simulink model "mpc_active_suspension_2020b"  (R2020b)
settings: Solver=FixedStepAuto  StartTime=0.0  StopTime=10  FixedStep=0.001  MaxStep=0.001  RelTol=1e-3
undefined symbols (not defined in the file): A, B, C, D, kw, Q, R, sigbuilder_block, T
libraries: simulink x1, dsparch4 x1
settings Model: Creator=ku53058  LastModifiedBy=11508
settings DataIOCC: ReturnWorkspaceOutputs=off
settings OptimizationCC: LifeSpan=inf
settings DebuggingCC: ArithmeticOperatorsInVariantConditions=warning
settings SFSimCC: SimUseLocalCustomCode=off  CustomCodeUndefinedFunction=UseInterfaceOnly
settings RTWCC: RTWUseLocalCustomCode=off
settings CodeAppCC: StateflowObjectComments=on

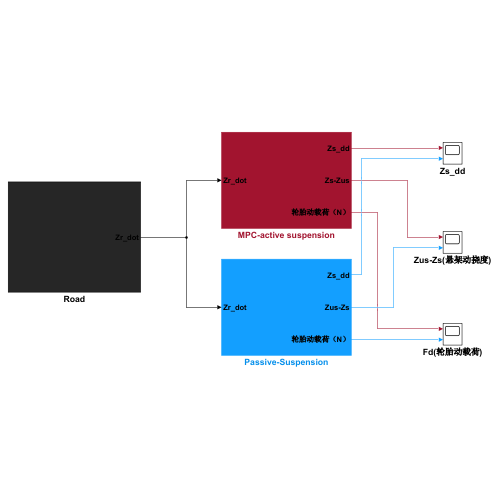
[thumbnail: Simulink's stored preview of the top-level diagram]
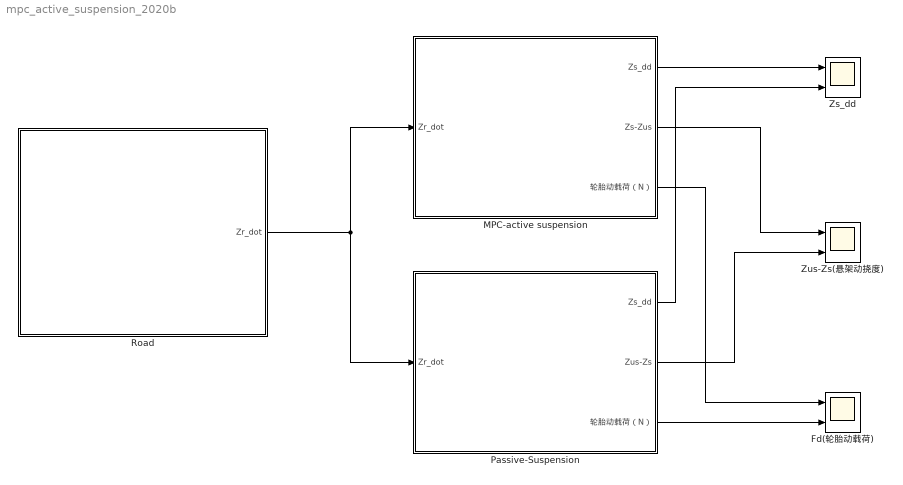
== system mpc_active_suspension_2020b ==
  Fd(轮胎动载荷) : Scope  NumInputPorts=2
  MPC-active suspension : Subsystem
  Passive-Suspension : Subsystem
  Road : Subsystem
  Zs_dd : Scope  NumInputPorts=2
  Zus-Zs(悬架动挠度) : Scope  NumInputPorts=2
  wires:
  MPC-active suspension/3(轮胎动载荷（N）) -> Fd(轮胎动载荷)/1
  MPC-active suspension/2(Zs-Zus) -> Zus-Zs(悬架动挠度)/1
  Road/1(Zr_dot) -> MPC-active suspension/1(Zr_dot), Passive-Suspension/1(Zr_dot)
  MPC-active suspension/1(Zs_dd) -> Zs_dd/1
  Passive-Suspension/3(轮胎动载荷（N）) -> Fd(轮胎动载荷)/2
  Passive-Suspension/2(Zus-Zs) -> Zus-Zs(悬架动挠度)/2
  Passive-Suspension/1(Zs_dd) -> Zs_dd/2

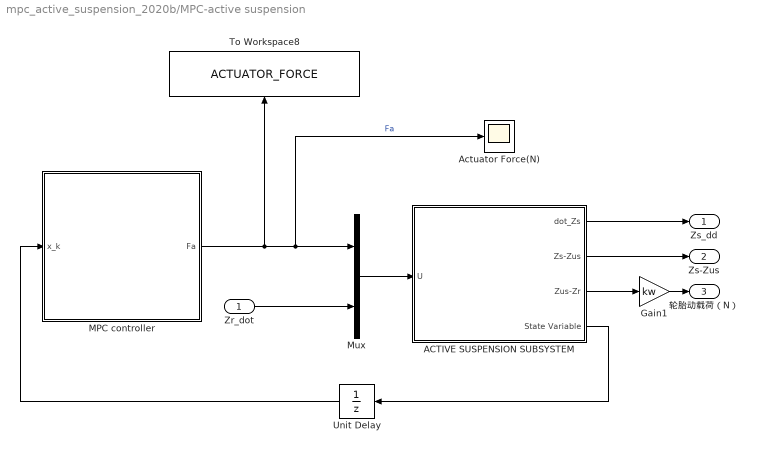
== system mpc_active_suspension_2020b/MPC-active suspension ==
  Zr_dot : Inport
  ACTIVE SUSPENSION SUBSYSTEM : Subsystem
  Actuator Force(N) : Scope
  Gain1 : Gain  Gain=kw
  MPC controller : Subsystem
  Mux : Mux  Inputs=2
  To Workspace8 : ToWorkspace  VariableName=ACTUATOR_FORCE  SampleTime=-1
  Unit Delay : UnitDelay  SampleTime=-1  HasFrameUpgradeWarning=on
  Zs_dd : Outport
  Zs-Zus : Outport  Port=2
  轮胎动载荷（N） : Outport  Port=3
  wires:
  Mux/1 -> ACTIVE SUSPENSION SUBSYSTEM/1(U)
  MPC controller/1(Fa) -> Mux/1, Actuator Force(N)/1, To Workspace8/1  "Fa"
  ACTIVE SUSPENSION SUBSYSTEM/2(Zs-Zus) -> Zs-Zus/1
  ACTIVE SUSPENSION SUBSYSTEM/3(Zus-Zr) -> Gain1/1
  Gain1/1 -> 轮胎动载荷（N）/1
  ACTIVE SUSPENSION SUBSYSTEM/1(dot_Zs) -> Zs_dd/1
  Zr_dot/1 -> Mux/2
  ACTIVE SUSPENSION SUBSYSTEM/4(State Variable) -> Unit Delay/1
  Unit Delay/1 -> MPC controller/1(x_k)

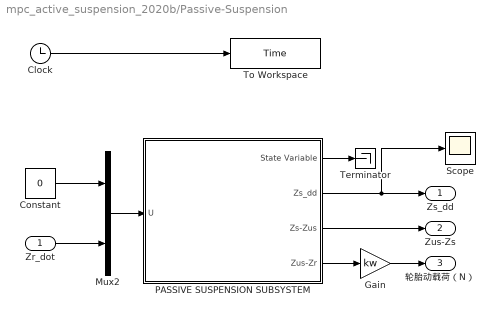
== system mpc_active_suspension_2020b/Passive-Suspension ==
  Zr_dot : Inport
  Clock : Clock
  Constant : Constant  Value=0
  Gain : Gain  Gain=kw
  Mux2 : Mux  Inputs=2
  PASSIVE SUSPENSION SUBSYSTEM : Subsystem
  Scope : Scope
  Terminator : Terminator
  To Workspace : ToWorkspace  VariableName=Time  SampleTime=-1
  Zs_dd : Outport
  Zus-Zs : Outport  Port=2
  轮胎动载荷（N） : Outport  Port=3
  wires:
  Mux2/1 -> PASSIVE SUSPENSION SUBSYSTEM/1(U)
  PASSIVE SUSPENSION SUBSYSTEM/3(Zs-Zus) -> Zus-Zs/1
  PASSIVE SUSPENSION SUBSYSTEM/2(Zs_dd) -> Scope/1, Zs_dd/1
  Gain/1 -> 轮胎动载荷（N）/1
  PASSIVE SUSPENSION SUBSYSTEM/4(Zus-Zr) -> Gain/1
  Zr_dot/1 -> Mux2/2
  Constant/1 -> Mux2/1
  Clock/1 -> To Workspace/1
  PASSIVE SUSPENSION SUBSYSTEM/1(State Variable) -> Terminator/1

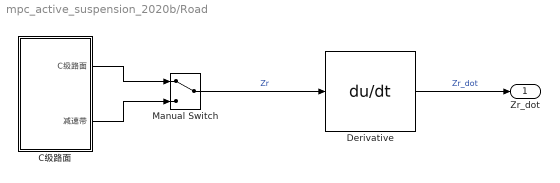
== system mpc_active_suspension_2020b/Road ==
  C级路面 : Subsystem
  Derivative : Derivative
  Manual Switch : ManualSwitch
  Zr_dot : Outport
  wires:
  Manual Switch/1 -> Derivative/1  "Zr"
  Derivative/1 -> Zr_dot/1  "Zr_dot"
  C级路面/2(减速带) -> Manual Switch/2
  C级路面/1(C级路面) -> Manual Switch/1

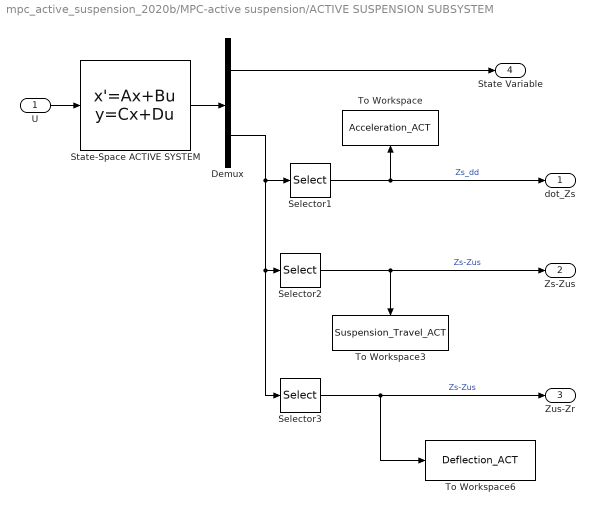
== system mpc_active_suspension_2020b/MPC-active suspension/ACTIVE SUSPENSION SUBSYSTEM ==
  U : Inport
  Demux : Demux  Outputs=[4 3]
  Selector1 : Selector  InputPortWidth=3  IndexOptions=Index vector (dialog)  Indices=[1]  OutputSizes=1
  Selector2 : Selector  InputPortWidth=3  IndexOptions=Index vector (dialog)  Indices=2  OutputSizes=1
  Selector3 : Selector  InputPortWidth=3  IndexOptions=Index vector (dialog)  Indices=3  OutputSizes=1
  State-Space ACTIVE SYSTEM : StateSpace  A=A  B=cat(2,B,E)  C=cat(1,eye(4), C)  D=cat(1,zeros(4,2),cat(2,D,T))  InitialCondition=0
  To Workspace : ToWorkspace  VariableName=Acceleration_ACT  SampleTime=-1
  To Workspace3 : ToWorkspace  VariableName=Suspension_Travel_ACT  SampleTime=-1
  To Workspace6 : ToWorkspace  VariableName=Deflection_ACT  SampleTime=-1
  dot_Zs : Outport
  Zs-Zus : Outport  Port=2
  Zus-Zr : Outport  Port=3
  State Variable : Outport  Port=4
  wires:
  Demux/1 -> State Variable/1
  State-Space ACTIVE SYSTEM/1 -> Demux/1
  Demux/2 -> Selector1/1, Selector3/1, Selector2/1
  Selector1/1 -> dot_Zs/1, To Workspace/1  "Zs_dd"
  Selector2/1 -> Zs-Zus/1, To Workspace3/1  "Zs-Zus"
  U/1 -> State-Space ACTIVE SYSTEM/1
  Selector3/1 -> To Workspace6/1, Zus-Zr/1  "Zs-Zus"

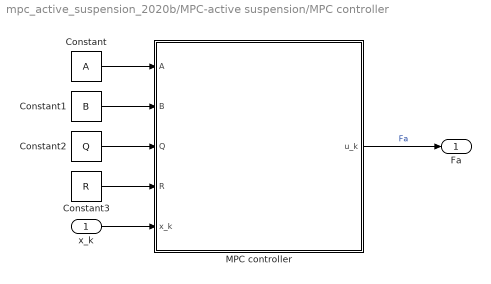
== system mpc_active_suspension_2020b/MPC-active suspension/MPC controller ==
  x_k : Inport
  Constant : Constant  Value=A  VectorParams1D=off
  Constant1 : Constant  Value=B  VectorParams1D=off
  Constant2 : Constant  Value=Q  VectorParams1D=off
  Constant3 : Constant  Value=R  VectorParams1D=off
  MPC controller : MATLAB Function  TreatAsAtomicUnit=on
  Fa : Outport
  wires:
  Constant/1 -> MPC controller/1(A)
  Constant2/1 -> MPC controller/3(Q)
  Constant3/1 -> MPC controller/4(R)
  x_k/1 -> MPC controller/5(x_k)
  Constant1/1 -> MPC controller/2(B)
  MPC controller/1(u_k) -> Fa/1  "Fa"

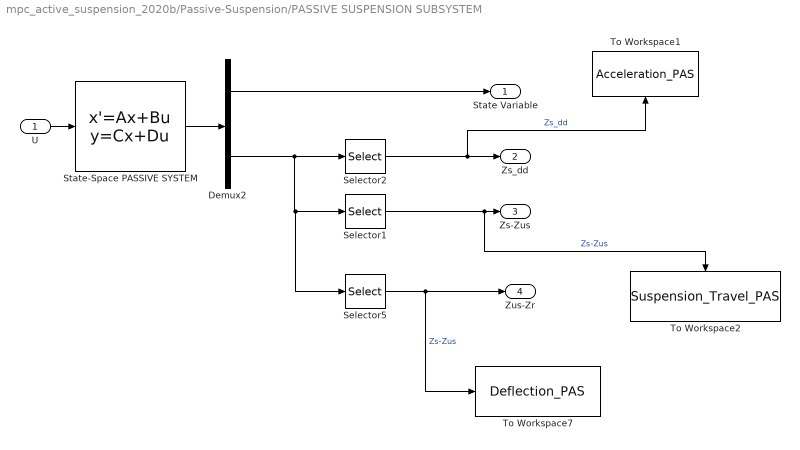
== system mpc_active_suspension_2020b/Passive-Suspension/PASSIVE SUSPENSION SUBSYSTEM ==
  U : Inport
  Demux2 : Demux  Outputs=[4 3]
  Selector1 : Selector  InputPortWidth=3  IndexOptions=Index vector (dialog)  Indices=2  OutputSizes=1
  Selector2 : Selector  InputPortWidth=3  IndexOptions=Index vector (dialog)  Indices=[1]  OutputSizes=1
  Selector5 : Selector  InputPortWidth=3  IndexOptions=Index vector (dialog)  Indices=3  OutputSizes=1
  State-Space PASSIVE SYSTEM : StateSpace  A=A  B=cat(2,B,E)  C=cat(1,eye(4), C)  D=cat(1,zeros(4,2),cat(2,D,T))  InitialCondition=0
  To Workspace1 : ToWorkspace  VariableName=Acceleration_PAS  SampleTime=-1
  To Workspace2 : ToWorkspace  VariableName=Suspension_Travel_PAS  SampleTime=-1
  To Workspace7 : ToWorkspace  VariableName=Deflection_PAS  SampleTime=-1
  State Variable : Outport
  Zs_dd : Outport  Port=2
  Zs-Zus : Outport  Port=3
  Zus-Zr : Outport  Port=4
  wires:
  State-Space PASSIVE SYSTEM/1 -> Demux2/1
  U/1 -> State-Space PASSIVE SYSTEM/1
  Demux2/1 -> State Variable/1
  Demux2/2 -> Selector5/1, Selector1/1, Selector2/1
  Selector2/1 -> To Workspace1/1, Zs_dd/1  "Zs_dd"
  Selector1/1 -> Zs-Zus/1, To Workspace2/1  "Zs-Zus"
  Selector5/1 -> To Workspace7/1, Zus-Zr/1  "Zs-Zus"

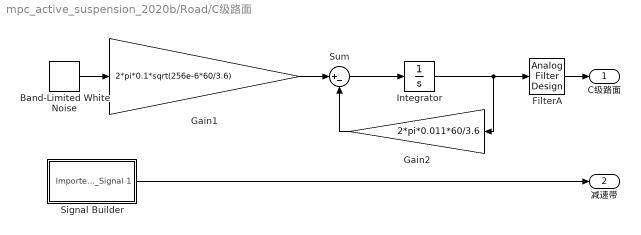
== system mpc_active_suspension_2020b/Road/C级路面 ==
  Band-Limited White Noise : simulink/Sources/Band-Limited White Noise  Cov=0.5  Ts=0.01  seed=[23341]
  FilterA : dsparch4/Analog Filter Design  method=Butterworth  filttype=Bandpass  N=4  Wlo=0.01*2*pi  Whi=20*2*pi  Rp=2  Rs=40
  Gain1 : Gain  Gain=2*pi*0.1*sqrt(256e-6*60/3.6)
  Gain2 : Gain  Gain=2*pi*0.011*60/3.6
  Integrator : Integrator
  Signal Builder : Subsystem  Tag=STV Subsys  LoadFcn=sigbuilder_block('load');  StartFcn=sigbuilder_block('start');  StopFcn=sigbuilder_block('stop');  ClipboardFcn=sigbuilder_block('clipboard');  mask(Sigbuilder block){tuvar=[0:10]}
      mask help: Simulink:masks:SigbuilderBlock_MD
      mask init:
      | if ~strcmp(get_param(bdroot(gcbh),'SimulationStatus'),'stopped') tuvar = sigbuilder_block('maskInit'); end
      settings: CopyFcn=sigbuilder_block('copy');  DeleteFcn=sigbuilder_block('delete');  ModelCloseFcn=sigbuilder_block('modelClose');  PreSaveFcn=sigbuilder_block('preSave');  PauseFcn=sigbuilder_block('pause');  ContinueFcn=sigbuilder_block('continue');  NameChangeFcn=sigbuilder_block('namechange');  OpenFcn=sigbuilder_block('open',[476.5 112.5 550.5 400 ]);  CloseFcn=sigbuilder_block('close');
      mask Display: plot(0, 0, 100, 100,[2, 2, 32, 32, 2], [68, 8, 8, 68, 68],[32, 2], [38, 38], [32, 19, 2],[53, 60, 44], [32, 17, 17, 2],[16, 16, 31, 31]);txt = getActiveGroup(gcbh);text(2, 100, txt,'verticalAlignment', 'top');
  Sum : Sum  Inputs=|+-
  C级路面 : Outport  VectorParamsAs1DForOutWhenUnconnected=off
  减速带 : Outport  Port=2  VectorParamsAs1DForOutWhenUnconnected=off
  wires:
  Signal Builder/1(Imported_Signal 1) -> 减速带/1
  Gain1/1 -> Sum/1
  Sum/1 -> Integrator/1
  Band-Limited White Noise/1 -> Gain1/1
  Integrator/1 -> Gain2/1, FilterA/1
  Gain2/1 -> Sum/2
  FilterA/1 -> C级路面/1

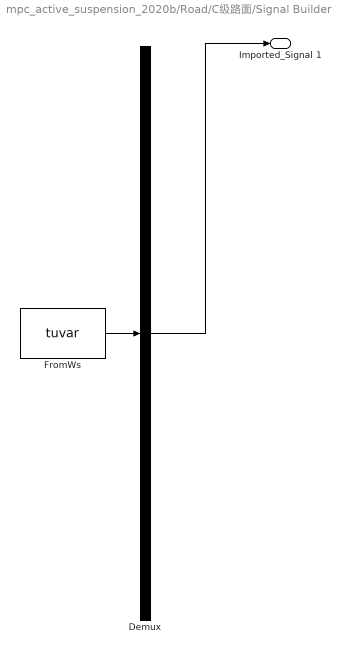
== system mpc_active_suspension_2020b/Road/C级路面/Signal Builder ==
  Demux : Demux  Tag=STV Demux  Outputs=1
      settings: DisplayOption=none
  FromWs : FromWorkspace  Tag=STV FromWs  VariableName=tuvar
      SigBuilderData=|
      | common.afterFinalStr = 'Extrapolate'
      | common.sampleTime = 0
      | dataSet.timeRange = [0 4]
      | dataSet.name = 'Sheet1'
      | sbobj.Groups.Name = 'Sheet1'
      | sbobj.Groups.Signals.Name = 'Imported_Signal 1'
      | sbobj.Groups.Signals.XData = [0 0.001 0.002 0.003 0.004 0.005 0.006 0.007 0.008 0.009 0.01 0.011 ... (4001 elements, 1x4001)]
      | sbobj.Groups.Signals.YData = [0 0 0 0 0 0 0 0 0 0 0 0 ... (4001 elements, 1x4001)]
      | sbobj.Groups.TimeRange = [0 4]
  Imported_Signal 1 : Outport  Tag=STV Outport  VectorParamsAs1DForOutWhenUnconnected=off
  wires:
  Demux/1 -> Imported_Signal 1/1
  FromWs/1 -> Demux/1

== matlab function mpc_active_suspension_2020b/MPC-active suspension/MPC controller/MPC controller ==
  data: A input; B input; Q input; R input; x_k input; u_k output
function u_k= fcn(A,B,Q,R,x_k)
n=size(A,1);   % A 是 n x n 矩阵, 得到 n
dt = 0.001;
I=eye(n);
A1 = I+A*dt;%离散化
B1 = dt*B;
p=size(B1,2);   % B 是 n x p 矩阵, 得到 p
Np = 10; %预测区间
[E,H]=MPC_Matrices(A1,B1,Q,R,Np,n,p); %求得E H矩阵
% 计算
u_k = Prediction(x_k,E,H,Np,p); %求得此步得uk


function  [E,H]=MPC_Matrices(A,B,Q,R,Np,n,p)  %算出E和H矩阵
B_hat=zeros(Np*n,Np*p); % 初始化 B_hat 矩阵, 这一步令它有 Np*n x Np*p 个 0
B_hat(1:n,1:p)=B; %
A_hat = A;
temp = A;
for i =1:(Np-1)  
rows = i*n+(1:n);  % 表示行 i = 1 -> row = n+1 : 2n  那 i = 1 : (Np-1) 行则 n+1 :  (Np-1)n + 1 : Np*n 
B_hat(rows,:)=[temp*B,B_hat(rows-n,1:end-p)]; %temp=A^i,  tempt*B并上上一大行（n行）去除最后一个元素（此元素p列）
temp =A*temp;
A_hat = [A_hat;temp];  % 并上新的矩阵
end
% 定义Q_ba和R_ba
Q_ba = kron(eye(Np),Q);
R_ba = kron(eye(Np),R); 
% 计算E, H
E=A_hat'*Q_ba*B_hat; % E: n x Np
H=B_hat'*Q_ba*B_hat+R_ba; % Np x Np
end 

function u_k= Prediction(x_k,E,H,Np,p) %二次规划求得最优的u_k
opts = optimoptions('quadprog','Algorithm','active-set');
x0 = zeros(Np*p,1);
max = 3000;
ub = kron(ones(Np,1),max);
lb = kron(ones(Np,1),-max);
f = E'*x_k;
U_k = quadprog(H,f,[],[],[],[],lb,ub,x0,opts);
u_k = U_k(1:p,1); % 取第一个结果
end
end
